simulink model "henon2d"  (Simulink 8.4)
settings: Solver=ode45  SolverMode=SingleTasking  StartTime=0.0  StopTime=100  RelTol=1e-3  AbsTol=1e-6
settings Model: Creator=The MathWorks Inc.  LastModifiedBy=gcampa  ExtModeTrigMode=oneshot  ExtModeArmWhenConnect=off
settings DataIOCC: ExternalInput=[]  InitialState=[]  LimitDataPoints=off  SaveOutput=off  SaveTime=off
settings OptimizationCC: BlockReduction=off  BooleanDataType=off  ExpressionDepthLimit=128  InitFltsAndDblsToZero=on
settings DebuggingCC: SaveWithParameterizedLinksMsg=none  SignalResolutionControl=TryResolveAllWithWarning  SolverPrmCheckMsg=none  MultiTaskDSMMsg=warning  MultiTaskCondExecSysMsg=none  IntegerOverflowMsg=none  FcnCallInpInsideContextMsg=EnableAllAsError  FrameProcessingCompatibilityMsg=error  StateNameClashWarn=none
settings HardwareCC: TargetUnknown=on
settings GRTTargetCC: TargetFcnLib=ansi_tfl_tmw.mat
settings ConfigComp: CovMetricSettings=dw  CovHtmlReporting=on  CovSaveCumulativeToWorkspaceVar=on  CovSaveSingleToWorkspaceVar=on  CovModelRefEnable=Off  CovExternalEMLEnable=off  CovSFcnEnable=off

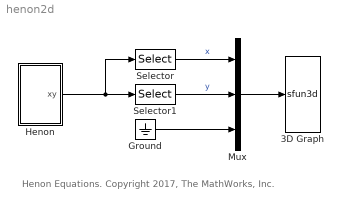
== system henon2d ==
  note: Henon Equations. Copyright 2017, The MathWorks, Inc.
  3D Graph : S-Function  LoadFcn=if exist('sfun3d','file'), sfun3d([],[],[],'LoadBlock'); end  FunctionName=sfun3d  Parameters=ax,T,np,cp,gd,ls,mk,mx,hd,tb  EnableBusSupport=off  mask(3D Graph){np=1, ax=[-2 2 [-1 1]/2 0 1], mx=2000, T=0.02, cp=[0 0 1], gd=on, hd=off, tb=off, ls=none, mk=.}
      mask prompts: np "Number of moving points (lines)"; ax "Range: [xmin xmax  ymin ymax zmin zmax]"; mx "Max number of points in each line"; T "Sampling Time"; cp "Camera position (use [0 0 1] for 2D XY view)"; gd "Grid (on|off)"; hd "HeadMarkers (on|off)"; tb "Toolbar (on|off)"; ls "LineStyle"; mk "LineMarker"
      mask help:
      | This block plots the position of several points in the XYZ space. The input contains the coordinates of all the points (x1,y1,z1,x2,y2,z2,...).
      | The number of moving points (lines), the XYZ ranges, sampling time, camera position, and grid (among other things) can be set as mask parameters.
      settings: CopyFcn=if exist('sfun3d','file'), sfun3d([],[],[],'CopyBlock'); end  DeleteFcn=if exist('sfun3d','file'), sfun3d([],[],[],'DeleteBlock'); end  NameChangeFcn=if exist('sfun3d','file'), sfun3d([],[],[],'NameChange'); end
      mask Help:
      | This block plots the position of several points in the XYZ space. The input contains the coordinates of all the points (x1,y1,z1,x2,y2,z2,...).
      | The number of moving points (lines), the XYZ ranges, sampling time, camera position, and grid (among other things) can be set as mask parameters.
      mask TypeOptions ls: - | -- | : | -. | none
      mask TypeOptions mk: none | . | + | o | * | x | square | diamond | v | ^ | > | < | pentagram | hexagram
      mask Display: plot([.05 .95 .95 .05 .05],[.45 .45 .95 .95 .45], 0.5+cos(0:0.1:2*pi)*0.3,0.7+sin(0:0.1:2*pi)*0.2)
  Ground : Ground
  Henon : Subsystem  mask(Henon System){a=1.4, b=0.3, xy0=[0 0], T=0.01}
      mask prompts: xy0 "Initial point p0 = [x0 y0]"; T "Sampling Time"
      mask help:
      | This autonomous system represents the henon equation:
      | xnew =  1 + y - a*x*x;  ynew =  b*x;
      | Parameters and initial state can be selected from the mask.
      mask Help:
      | This autonomous system represents the henon equation.
      | Parameters and initial state can be selected from the mask.
      | <p>
      | The system equations are:
      | xnew =  1 + y - a*x*x;
      | ynew =  b*x;
  Mux : Mux  Inputs=3
  Selector : Selector  InputPortWidth=2
  Selector1 : Selector  InputPortWidth=2  Indices=2
  wires:
  Henon/1(xy) -> Selector/1, Selector1/1
  Selector/1 -> Mux/1  "x"
  Selector1/1 -> Mux/2  "y"
  Ground/1 -> Mux/3
  Mux/1 -> 3D Graph/1

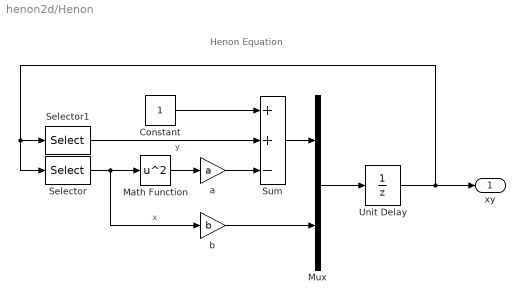
== system henon2d/Henon ==
  note: Henon Equation
  Constant : Constant
  Math Function : Math  Operator=square  SaturateOnIntegerOverflow=on
  Mux : Mux  Inputs=[1 1]
  Selector : Selector  InputPortWidth=2
  Selector1 : Selector  InputPortWidth=2  Indices=2
  Sum : Sum  Inputs=++-  SaturateOnIntegerOverflow=on  InputSameDT=on  OutDataTypeStr=Inherit: Same as first input
  Unit Delay : UnitDelay  InitialCondition=xy0  SampleTime=T
  a : Gain  Gain=a  SaturateOnIntegerOverflow=on  OutDataTypeStr=Inherit: Same as input  ParamDataTypeStr=Inherit: Same as input
  b : Gain  Gain=b  SaturateOnIntegerOverflow=on  OutDataTypeStr=Inherit: Same as input  ParamDataTypeStr=Inherit: Same as input
  xy : Outport
  wires:
  Math Function/1 -> a/1
  a/1 -> Sum/3
  Sum/1 -> Mux/1
  Constant/1 -> Sum/1
  Selector1/1 -> Sum/2  "y"
  Selector/1 -> Math Function/1, b/1  "x"
  b/1 -> Mux/2
  Mux/1 -> Unit Delay/1
  Unit Delay/1 -> xy/1, Selector1/1, Selector/1
